simulink model "fuzzyLogic"  (R2021a)
settings: Solver=ode23  StartTime=0.0  StopTime=0.2  RelTol=1e-6
values from neighbouring files (symbols this model uses):
  Ce = 0.96    [BCMotor_params.mat]    (also in p_3_6.m = 0.058; paragraph 3_3_1.mat = 0.153; paragraph 3_3_2.mat = 0.153; paragraph 3_3_3.mat = 0.153)
  Cm = 1.85    [BCMotor_params.mat]    (also in p_3_6.m = 0.057; paragraph 3_3_1.mat = 0.156; paragraph 3_3_2.mat = 0.156; paragraph 3_3_3.mat = 0.156)
  J = 2.02e-05    [BCMotor_params.mat]    (also in p_3_6.m = 8.4e-05; paragraph 3_3_1.mat = 0.000122; paragraph 3_3_2.mat = 0.000122; paragraph 3_3_3.mat = 0.000122)
  Ly = 0.86e-3    (= 0.00086)    [p_3_6.m]    (also in paragraph 3_3_1.mat = 0.0001; paragraph 3_3_2.mat = 0.0001; paragraph 3_3_3.mat = 0.0001; paragraph_3 5.mat = 0.0001)
  Ry = 0.71    [p_3_6.m]    (also in paragraph 3_3_1.mat = 0.34; paragraph 3_3_2.mat = 0.34; paragraph 3_3_3.mat = 0.34; paragraph_3 5.mat = 0.34)
libraries: fuzblock x1
settings Model: Creator=slagt  LastModifiedBy=slagt
settings DebuggingCC: UnderSpecifiedDimensionMsg=warning

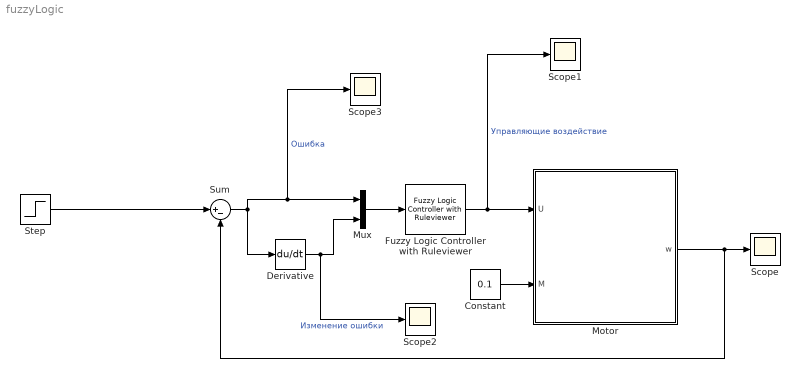
== system fuzzyLogic ==
  Constant : Constant  Value=0.1
  Derivative : Derivative
  Fuzzy Logic Controller with Ruleviewer : fuzblock/Fuzzy Logic  Controller  with Ruleviewer  fismatrix=fuzzy  Ts=2
  Motor : Subsystem
  Mux : Mux  Inputs=2
  Scope{,1..3} (4 alike) : Scope
  Step : Step  Time=0  SampleTime=0
  Sum : Sum  Inputs=|+-
  wires:
  Step/1 -> Sum/1
  Constant/1 -> Motor/2(M)
  Motor/1(w) -> Sum/2, Scope/1
  Fuzzy Logic Controller with Ruleviewer/1 -> Scope1/1, Motor/1(U)  "Управляющие воздействие"
  Mux/1 -> Fuzzy Logic Controller with Ruleviewer/1
  Sum/1 -> Scope3/1, Mux/1, Derivative/1  "Ошибка"
  Derivative/1 -> Scope2/1, Mux/2  "Изменение ошибки"

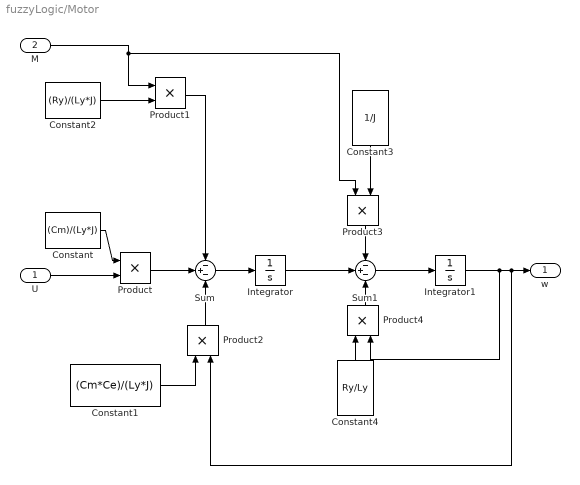
== system fuzzyLogic/Motor ==
  U : Inport
  M : Inport  Port=2
  Constant : Constant  Value=(Cm)/(Ly*J)
  Constant1 : Constant  Value=(Cm*Ce)/(Ly*J)
  Constant2 : Constant  Value=(Ry)/(Ly*J)
  Constant3 : Constant  Value=1/J
  Constant4 : Constant  Value=Ry/Ly
  Integrator : Integrator
  Integrator1 : Integrator
  Product{,1..4} (5 alike) : Product
  Sum : Sum  Inputs=-+-
  Sum1 : Sum  Inputs=-+-
  w : Outport
  wires:
  U/1 -> Product/2
  Product/1 -> Sum/2
  M/1 -> Product1/1, Product3/1
  Product1/1 -> Sum/1
  Constant2/1 -> Product1/2
  Product2/1 -> Sum/3
  Sum/1 -> Integrator/1
  Integrator/1 -> Sum1/2
  Sum1/1 -> Integrator1/1
  Product3/1 -> Sum1/1
  Product4/1 -> Sum1/3
  Integrator1/1 -> Product4/2, Product2/2, w/1
  Constant/1 -> Product/1
  Constant1/1 -> Product2/1
  Constant3/1 -> Product3/2
  Constant4/1 -> Product4/1
